simulink model "currentvelocity"  (R2023a)
settings: Solver=FixedStepAuto  StartTime=0.0  StopTime=120  FixedStep=0.03  RelTol=1e-3
values from neighbouring files (symbols this model uses):
  b_1 = 51.0314    [modelsetup.m]
  b_2 = -13.8341    [modelsetup.m]
  EPSILON = 0.005    [modelsetup.m]
  F_kinetic = 8.1003    [modelsetup.m]
  F_static = 10.4160    (= 10.416)    [modelsetup.m]
  J = 9.1617    [modelsetup.m]
  K_t = 0.124 * 120    (= 14.88)    [modelsetup.m]
libraries: simulink x1
settings Model: Creator=yunzh  LastModifiedBy=yunzh

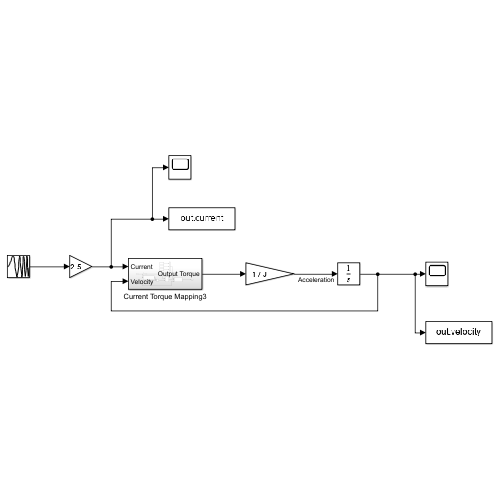
[thumbnail: Simulink's stored preview of the top-level diagram]
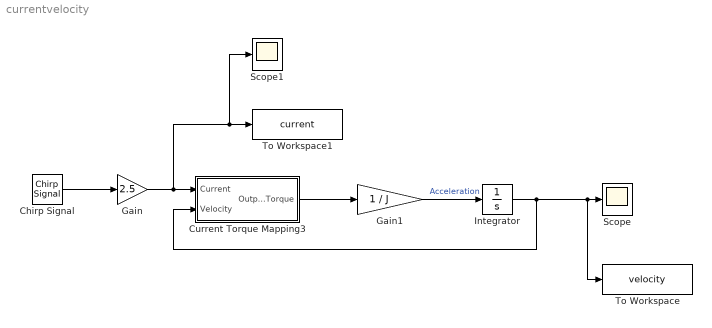
== system currentvelocity ==
  Chirp Signal : simulink/Sources/Chirp Signal  f1=0  T=120  f2=25
  Current Torque Mapping3 : Subsystem
  Gain : Gain  Gain=2.5
  Gain1 : Gain  Gain=1 / J
  Integrator : Integrator
  Scope : Scope
  Scope1 : Scope
  To Workspace : ToWorkspace  VariableName=velocity  SaveFormat=Timeseries  SampleTime=-1
  To Workspace1 : ToWorkspace  VariableName=current  SaveFormat=Timeseries  SampleTime=-1
  wires:
  Current Torque Mapping3/1(Output Torque) -> Gain1/1
  Gain1/1 -> Integrator/1  "Acceleration"
  Integrator/1 -> To Workspace/1, Scope/1, Current Torque Mapping3/2(Velocity)
  Chirp Signal/1 -> Gain/1
  Gain/1 -> Scope1/1, To Workspace1/1, Current Torque Mapping3/1(Current)

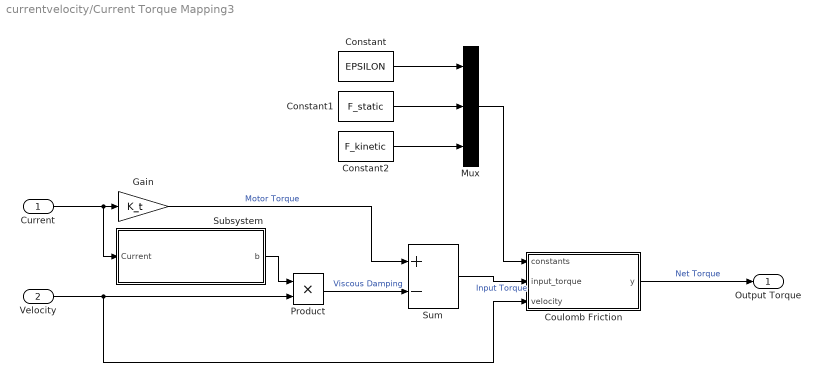
== system currentvelocity/Current Torque Mapping3 ==
  Current : Inport
  Velocity : Inport  Port=2
  Constant : Constant  Value=EPSILON
  Constant1 : Constant  Value=F_static
  Constant2 : Constant  Value=F_kinetic
  Coulomb Friction : MATLAB Function  TreatAsAtomicUnit=on
  Gain : Gain  Gain=K_t
  Mux : Mux  Inputs=3
  Product : Product
  Subsystem : Subsystem
  Sum : Sum  Inputs=+-
  Output Torque : Outport
  wires:
  Constant1/1 -> Mux/2
  Gain/1 -> Sum/1  "Motor Torque"
  Mux/1 -> Coulomb Friction/1(constants)
  Sum/1 -> Coulomb Friction/2(input_torque)  "Input Torque"
  Constant/1 -> Mux/1
  Constant2/1 -> Mux/3
  Current/1 -> Subsystem/1(Current), Gain/1
  Velocity/1 -> Product/2, Coulomb Friction/3(velocity)
  Coulomb Friction/1(y) -> Output Torque/1  "Net Torque"
  Product/1 -> Sum/2  "Viscous Damping"
  Subsystem/1(b) -> Product/1

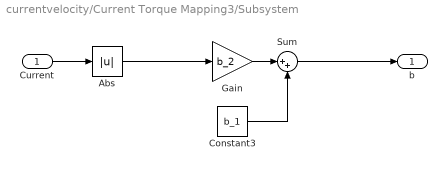
== system currentvelocity/Current Torque Mapping3/Subsystem ==
  Current : Inport
  Abs : Abs  SaturateOnIntegerOverflow=off
  Constant3 : Constant  Value=b_1
  Gain : Gain  Gain=b_2
  Sum : Sum  Inputs=|++
  b : Outport
  wires:
  Current/1 -> Abs/1
  Gain/1 -> Sum/1
  Sum/1 -> b/1
  Constant3/1 -> Sum/2
  Abs/1 -> Gain/1

== matlab function currentvelocity/Current Torque Mapping3/Coulomb Friction ==
  data: constants input; input_torque input; velocity input; y output
function y = fcn(constants, input_torque, velocity)
    EPSILON = constants(1);
    F_stat = constants(2);
    F_c = constants(3);


    if abs(velocity) < EPSILON % no motion
        if abs(input_torque) < abs(F_stat) % insufficient torque
            y = 0;
            return
        end

        % reduce torque by static friction
        static_friction = -1 * sign(input_torque) * F_stat;
        y = input_torque + static_friction;
        return
    end
    
    % reduce torque by dynamic friction
    dynamic_friction = -1 * sign(velocity) * F_c;
    y = input_torque + dynamic_friction;
end
